simulink model "nms_3Dmodel_inv_wAnkleCPG"  (R2016b)
settings: Solver=ode3  StartTime=0.0  StopTime=tend  FixedStep=ts  RelTol=1e-3  EnableMultiTasking=on
InitFcn:
  | runScripts_inv;
values from neighbouring files (symbols this model uses):
  c = 0.05    [IID_nms_MechInit.m]    (also in nms_MechInit.m)
  c_jointstop = 0.3 / (pi/180)    (= 17.1887338539)    [IID_nms_MechInit.m]    (also in nms_MechInit.m)
  CPG_On = 1    [setCPGPar.m]    (also in setCPGPar_inv.m)
  CtrlPar_FP = [alpha0 alpha_cd alpha_cv]    [setCtrlPar.m]
  CtrlPar_FP_R = [R_hipR0 R_hipR_cd R_hipR_cv]    [setCtrlPar.m]
  CtrlPar_LL = l_clr    [setCtrlPar.m]
  CtrlPar_St = [StPreStim St_M1 St_M2 St_M3 St_M4 St_M5 St_M11]    [setCtrlPar.m]
  CtrlPar_St_R = [R_StPreStim R_St_M1 R_St_M3 R_St_M4]    [setCtrlPar.m]
  CtrlPar_Sw = [SwPreStim SwPhasePari SwPhaseParii SwCtrlPar_H SwCtrlPar_A      SwCtrlPar_Ki SwCtrlPar_Kii SwCtrlPar_Kiii SwCtrlPar_StP]    [setCtrlPar.m]
  CtrlPar_Sw_R = [R_SwPreStim R_Sw_M6]    [setCtrlPar.m]
  CtrlPar_theta0 = parBlCtrl(1)      *1*pi/180    [setCtrlPar.m]
  CtrlPar_Tr = [Tr_St_sup Tr_Sw]    [setCtrlPar.m]
  CtrlPar_Tr_R = [R_Tr_St_sup R_Tr_Sw]    [setCtrlPar.m]
  eref = 0.04    [IID_nms_MechInit.m]    (also in nms_MechInit.m)
  FmaxBFSH = 350    [nms_MechInit.m]
  FmaxGAS = 1500    [IID_nms_MechInit.m]    (also in nms_MechInit.m)
  FmaxGLU = 1500    [IID_nms_MechInit.m]    (also in nms_MechInit.m)
  FmaxHAB = 3000    [nms_MechInit.m]
  FmaxHAD = 4500    [nms_MechInit.m]
  FmaxHAM = 3000    [IID_nms_MechInit.m]    (also in nms_MechInit.m)
  FmaxHFL = 2000    [IID_nms_MechInit.m]    (also in nms_MechInit.m)
  FmaxRF = 1200    [nms_MechInit.m]
  FmaxSOL = 4000    [IID_nms_MechInit.m]    (also in nms_MechInit.m)
  FmaxTA = 800    [IID_nms_MechInit.m]    (also in nms_MechInit.m)
  FmaxVAS = 6000    [IID_nms_MechInit.m]    (also in nms_MechInit.m)
  init_a_tgt = 70*pi/180    (= 1.2217304764)    [setInitPar.m]
  init_a_tgtR = 90*pi/180    (= 1.57079632679)    [setInitPar.m]
  K = 5    [IID_nms_MechInit.m]    (also in nms_MechInit.m)
  leg_l = [D12_T D12_S]    [nms_MechInit.m]
  LongDelay = 0.020    (= 0.02)    [IID_setCtrlPar.m]    (also in nms_MechInit.m = 0.01)
  LongLoopDelay = 0.030    (= 0.03)    [nms_MechInit.m]
  loptBFSH = 0.12    [nms_MechInit.m]
  loptGAS = 0.05    [IID_nms_MechInit.m]    (also in nms_MechInit.m)
  loptGLU = 0.11    [IID_nms_MechInit.m]    (also in nms_MechInit.m)
  loptHAB = 0.09    [nms_MechInit.m]
  loptHAD = 0.10    (= 0.1)    [nms_MechInit.m]
  loptHAM = 0.10    (= 0.1)    [IID_nms_MechInit.m]    (also in nms_MechInit.m)
  loptHFL = 0.11    [IID_nms_MechInit.m]    (also in nms_MechInit.m)
  loptRF = 0.08    [nms_MechInit.m]
  loptSOL = 0.04    [IID_nms_MechInit.m]    (also in nms_MechInit.m)
  loptTA = 0.06    [IID_nms_MechInit.m]    (also in nms_MechInit.m)
  loptVAS = 0.08    [IID_nms_MechInit.m]    (also in nms_MechInit.m)
  lslackBFSH = 0.10    (= 0.1)    [nms_MechInit.m]
  lslackGAS = 0.40    (= 0.4)    [IID_nms_MechInit.m]    (also in nms_MechInit.m)
  lslackGLU = 0.13    [IID_nms_MechInit.m]    (also in nms_MechInit.m)
  lslackHAB = 0.07    [nms_MechInit.m]
  lslackHAD = 0.18    [nms_MechInit.m]
  lslackHAM = 0.31    [IID_nms_MechInit.m]    (also in nms_MechInit.m)
  lslackHFL = 0.10    (= 0.1)    [IID_nms_MechInit.m]    (also in nms_MechInit.m)
  lslackRF = 0.35    [nms_MechInit.m]
  lslackSOL = 0.26    [IID_nms_MechInit.m]    (also in nms_MechInit.m)
  lslackTA = 0.24    [IID_nms_MechInit.m]    (also in nms_MechInit.m)
  lslackVAS = 0.23    [IID_nms_MechInit.m]    (also in nms_MechInit.m)
  massBFSH = 2    [nms_MechInit.m]
  massGAS = 0.45    [IID_nms_MechInit.m]    (also in nms_MechInit.m)
  massGLU = 1.4    [IID_nms_MechInit.m]    (also in nms_MechInit.m)
  massHAB = 1.145    [nms_MechInit.m]
  massHAD = 1.91    [nms_MechInit.m]
  massHAM = 1.82    [IID_nms_MechInit.m]    (also in nms_MechInit.m)
  massHFL = 1.87    [IID_nms_MechInit.m]    (also in nms_MechInit.m)
  massRF = 1    [nms_MechInit.m]
  massSOL = 1.36    [IID_nms_MechInit.m]    (also in nms_MechInit.m)
  massTA = 0.29    [IID_nms_MechInit.m]    (also in nms_MechInit.m)
  massVAS = 2.91    [IID_nms_MechInit.m]    (also in nms_MechInit.m)
  MidDelay = 0.010    (= 0.01)    [IID_setCtrlPar.m]    (also in nms_MechInit.m = 0.005)
  N = 1.5    [IID_nms_MechInit.m]    (also in cmaes_parfor.m = size(x,1); nms_MechInit.m)
  phi12_LowLimit = 70*pi/180    (= 1.2217304764)    [IID_nms_MechInit.m]    (also in nms_MechInit.m)
  phi12_UpLimit = 130*pi/180    (= 2.26892802759)    [IID_nms_MechInit.m]    (also in nms_MechInit.m)
  phi23_UpLimit = 175*pi/180    (= 3.05432619099)    [IID_nms_MechInit.m]    (also in nms_MechInit.m)
  phi34_UpLimit = 230*pi/180    (= 4.01425727959)    [IID_nms_MechInit.m]    (also in nms_MechInit.m)
  phi34R_LowLimit = -15*pi/180    (= -0.261799387799)    [nms_MechInit.m]
  phi34R_UpLimit = 50*pi/180    (= 0.872664625997)    [nms_MechInit.m]
  phimaxGASa = 110*pi/180    (= 1.91986217719)    [IID_nms_MechInit.m]    (also in nms_MechInit.m = 1.74532925199)
  phimaxGASk = 140*pi/180    (= 2.44346095279)    [IID_nms_MechInit.m]    (also in nms_MechInit.m)
  phimaxRFk = 165*pi/180    (= 2.87979326579)    [nms_MechInit.m]
  phimaxSOL = 110*pi/180    (= 1.91986217719)    [IID_nms_MechInit.m]    (also in nms_MechInit.m = 1.74532925199)
  phimaxTA = 80*pi/180    (= 1.3962634016)    [IID_nms_MechInit.m]    (also in nms_MechInit.m)
  phimaxVAS = 165*pi/180    (= 2.87979326579)    [IID_nms_MechInit.m]    (also in nms_MechInit.m)
  phirefBFSH = 160*pi/180    (= 2.79252680319)    [nms_MechInit.m]
  phirefGASa = 80*pi/180    (= 1.3962634016)    [IID_nms_MechInit.m]    (also in nms_MechInit.m)
  phirefGASk = 165*pi/180    (= 2.87979326579)    [IID_nms_MechInit.m]    (also in nms_MechInit.m)
  phirefGLU = 150*pi/180    (= 2.61799387799)    [IID_nms_MechInit.m]    (also in nms_MechInit.m = 2.09439510239)
  phirefHAB = 10*pi/180    (= 0.174532925199)    [nms_MechInit.m]
  phirefHAD = 15*pi/180    (= 0.261799387799)    [nms_MechInit.m]
  phirefHAMh = 155*pi/180    (= 2.70526034059)    [IID_nms_MechInit.m]    (also in nms_MechInit.m = 2.61799387799)
  phirefHAMk = 180*pi/180    (= 3.14159265359)    [IID_nms_MechInit.m]    (also in nms_MechInit.m)
  phirefHFL = 180*pi/180    (= 3.14159265359)    [IID_nms_MechInit.m]    (also in nms_MechInit.m = 2.79252680319)
  phirefRFh = 170*pi/180    (= 2.96705972839)    [nms_MechInit.m]
  phirefRFk = 125*pi/180    (= 2.18166156499)    [nms_MechInit.m]
  phirefSOL = 80*pi/180    (= 1.3962634016)    [IID_nms_MechInit.m]    (also in nms_MechInit.m = 1.57079632679)
  phirefTA = 110*pi/180    (= 1.91986217719)    [IID_nms_MechInit.m]    (also in nms_MechInit.m)
  phirefVAS = 125*pi/180    (= 2.18166156499)    [IID_nms_MechInit.m]    (also in nms_MechInit.m = 2.09439510239)
  phiScaleGASa = acos(rGASamin/rGASamax)/(phiminGASa-phimaxGASa)    [nms_MechInit.m]
  phiScaleGASk = acos(rGASkmin/rGASkmax)/(phiminGASk-phimaxGASk)    [nms_MechInit.m]
  phiScaleRFk = acos(rRFkmin/rRFkmax)/(phiminRFk-phimaxRFk)    [nms_MechInit.m]
  phiScaleSOL = acos(rSOLmin/rSOLmax)/(phiminSOL-phimaxSOL)    [nms_MechInit.m]
  phiScaleTA = acos(rTAmin/rTAmax)/(phiminTA-phimaxTA)    [nms_MechInit.m]
  phiScaleVAS = acos(rVASmin/rVASmax)/(phiminVAS-phimaxVAS)    [nms_MechInit.m]
  rBFSH = 0.04    [nms_MechInit.m]
  rGASamax = 0.06    [nms_MechInit.m]
  rGASkmax = 0.05    [nms_MechInit.m]
  rGLU = 0.10    (= 0.1)    [IID_nms_MechInit.m]    (also in nms_MechInit.m = 0.08)
  rHAB = 0.06    [nms_MechInit.m]
  rHAD = 0.03    [nms_MechInit.m]
  rHAMh = 0.08    [IID_nms_MechInit.m]    (also in nms_MechInit.m)
  rHAMk = 0.05    [IID_nms_MechInit.m]    (also in nms_MechInit.m)
  rHFL = 0.10    (= 0.1)    [IID_nms_MechInit.m]    (also in nms_MechInit.m = 0.08)
  rhoBFSH = 0.7    [nms_MechInit.m]
  rhoGASa = 0.7    [IID_nms_MechInit.m]    (also in nms_MechInit.m)
  rhoGASk = 0.7    [IID_nms_MechInit.m]    (also in nms_MechInit.m)
  rhoGLU = 0.5    [IID_nms_MechInit.m]    (also in nms_MechInit.m)
  rhoHAB = 0.7    [nms_MechInit.m]
  rhoHAD = 1    [nms_MechInit.m]
  rhoHAMh = 0.7    [IID_nms_MechInit.m]    (also in nms_MechInit.m = 0.5)
  rhoHAMk = 0.7    [IID_nms_MechInit.m]    (also in nms_MechInit.m = 0.5)
  rhoHFL = 0.5    [IID_nms_MechInit.m]    (also in nms_MechInit.m)
  rhoRFh = 0.3    [nms_MechInit.m]
  rhoRFk = 0.5    [nms_MechInit.m]
  rhoSOL = 0.5    [IID_nms_MechInit.m]    (also in nms_MechInit.m)
  rhoTA = 0.7    [IID_nms_MechInit.m]    (also in nms_MechInit.m)
  ... (+55 more)
libraries: simulink_extras x30, nmc x30, simulink x22, NMCCPG_Library x13, powerlib_meascontrol x5
(part 2 of 12)

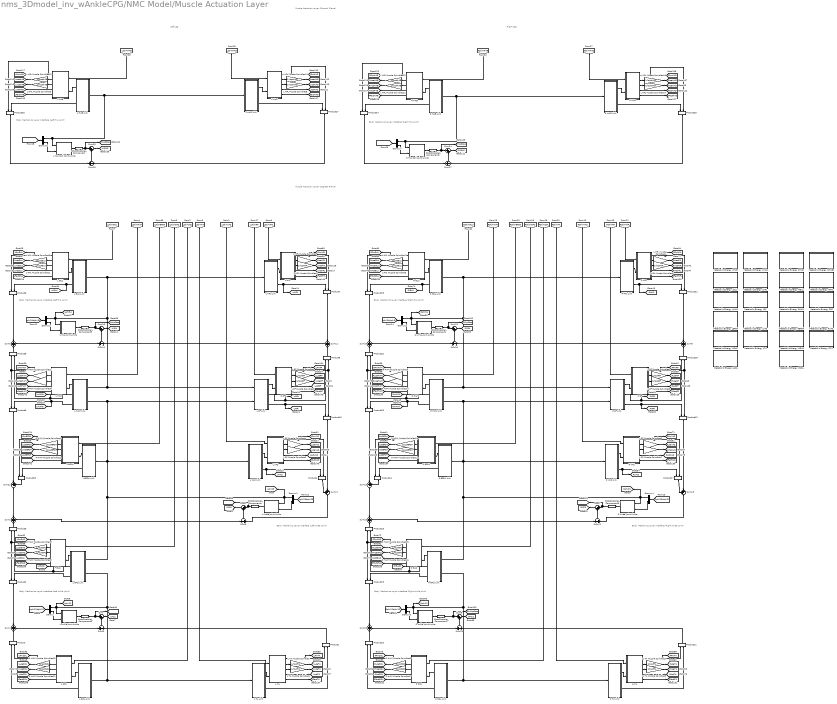
== system nms_3Dmodel_inv_wAnkleCPG/NMC Model/Muscle Actuation Layer ==
  note: Muscle Actuation Layer
      | (Coronal Plane)
  note: Right Leg
  note: Body Mechanics Layer
      | Interface (Right Hip Joint)
  note: Body Mechanics Layer
      | Interface (Left Hip Joint)
  note: Left Leg
  note: Body Mechanics Layer
      | Interface (Right Ankle Joint)
  note: Body Mechanics Layer
      | Interface (Right Knee Joint)
  note: Body Mechanics Layer
      | Interface (Right Hip Joint)
  note: Body Mechanics Layer
      | Interface (Left Ankle Joint)
  note: Body Mechanics Layer
      | Interface (Left Knee Joint)
  note: Body Mechanics Layer
      | Interface (Left Hip Joint)
  note: Muscle Actuation Layer
      | (Sagittal Plane)
  Demux{,1..7} (8 alike) : Demux  Outputs=2
  F GAS : Subsystem
  GotoDisabler_Component{,1..7} (8 alike) : nmc/GotoDisabler_Component  GotoTag=DisableNMC_JointLimits
  L Ankle Joint Limits : Subsystem
  L BFSH : Subsystem
  L BFSH Link : Subsystem
  L GAS Link : Subsystem
  L GLU : Subsystem
  L GLU Link : Subsystem
  L HAB : Subsystem
  L HAB Link : Subsystem
  L HAD : Subsystem
  L HAD Link : Subsystem
  L HAM : Subsystem
  L HAM Link : Subsystem
  L HFL : Subsystem
  L HFL Muscle Spindles{,1,4..5} (4 alike) : Gain  Gain=1/loptHFL
  L HFL Muscle Spindles{9..10,12..13} (4 alike) : Gain  Gain=1/loptHAB
  L HFL Muscle Spindles{8,11,14..15} (4 alike) : Gain  Gain=1/loptHAD
  L HFL Muscle Spindles{2..3,6..7} (4 alike) : Gain  Gain=1/loptGLU
  L HFL Link : Subsystem
  L Hip Joint Limits : Subsystem
  L Hip Roll Joint Limits : Subsystem
  L Knee Joint Limits : Subsystem
  L RF Muscle Spindles{,1..3} (4 alike) : Gain  Gain=1/loptRF
  L RF Muscle Spindles{4..7} (4 alike) : Gain  Gain=1/loptVAS
  L RF Link : Subsystem
  L SOL : Subsystem
  L SOL Link : Subsystem
  L TA : Subsystem
  L TA Muscle Spindles{,1..3} (4 alike) : Gain  Gain=1/loptTA
  L TA Link : Subsystem
  L VAS : Subsystem
  L VAS Link : Subsystem
  Metabolic Energy LBFSH : Subsystem  mask{side='L', muscle='BFSH'}
      mask prompts: side "What Side (R/L)?"; muscle "What Muscle?"
      mask init:
      | blk = gcb;
      | 
      | set_param([gcb '/From1'],'GotoTag',[side,'Act',muscle]);
      | set_param([gcb '/From2'],'GotoTag',[side,'Stim',muscle]);
      | set_param([gcb '/From3'],'GotoTag',[side,'Lce',muscle]);
      | set_param([gcb '/From4'],'GotoTag',[side,'Vce',muscle]);
      | set_param([gcb '/From5'],'GotoTag',[side,'Fm',muscle]);
      | set_param([gcb '/From6'],'GotoTag',[side,'Fact',muscle]);
      | 
      | set_param([gcb '/Goto1'],'GotoTag',[side,'Energy',muscle]);
      | 
      | set_param([gcb '/Constant'],'Value',['lopt',muscle]);
      | set_param([gcb '/Constant1'],'Value',['mass',muscle]);
      | set_param([gcb '/Constant2'],'Value',['t1f',muscle]);
  Metabolic Energy LGAS : Subsystem  mask{side='L', muscle='GAS'}
      mask prompts: side "What Side (R/L)?"; muscle "What Muscle?"
      mask init: same as nms_3Dmodel_inv_wAnkleCPG/NMC Model/Muscle Actuation Layer/Metabolic Energy LBFSH
  Metabolic Energy LGLU : Subsystem  mask{side='L', muscle='GLU'}
      mask prompts: side "What Side (R/L)?"; muscle "What Muscle?"
      mask init: same as nms_3Dmodel_inv_wAnkleCPG/NMC Model/Muscle Actuation Layer/Metabolic Energy LBFSH
  Metabolic Energy LHAB : Subsystem  mask{side='L', muscle='HAB'}
      mask prompts: side "What Side (R/L)?"; muscle "What Muscle?"
      mask init: same as nms_3Dmodel_inv_wAnkleCPG/NMC Model/Muscle Actuation Layer/Metabolic Energy LBFSH
  Metabolic Energy LHAD : Subsystem  mask{side='L', muscle='HAD'}
      mask prompts: side "What Side (R/L)?"; muscle "What Muscle?"
      mask init: same as nms_3Dmodel_inv_wAnkleCPG/NMC Model/Muscle Actuation Layer/Metabolic Energy LBFSH
  Metabolic Energy LHAM : Subsystem  mask{side='L', muscle='HAM'}
      mask prompts: side "What Side (R/L)?"; muscle "What Muscle?"
      mask init: same as nms_3Dmodel_inv_wAnkleCPG/NMC Model/Muscle Actuation Layer/Metabolic Energy LBFSH
  Metabolic Energy LHFL : Subsystem  mask{side='L', muscle='HFL'}
      mask prompts: side "What Side (R/L)?"; muscle "What Muscle?"
      mask init: same as nms_3Dmodel_inv_wAnkleCPG/NMC Model/Muscle Actuation Layer/Metabolic Energy LBFSH
  Metabolic Energy LRF : Subsystem  mask{side='L', muscle='RF'}
      mask prompts: side "What Side (R/L)?"; muscle "What Muscle?"
      mask init: same as nms_3Dmodel_inv_wAnkleCPG/NMC Model/Muscle Actuation Layer/Metabolic Energy LBFSH
  Metabolic Energy LSOL : Subsystem  mask{side='L', muscle='SOL'}
      mask prompts: side "What Side (R/L)?"; muscle "What Muscle?"
      mask init: same as nms_3Dmodel_inv_wAnkleCPG/NMC Model/Muscle Actuation Layer/Metabolic Energy LBFSH
  Metabolic Energy LTA : Subsystem  mask{side='L', muscle='TA'}
      mask prompts: side "What Side (R/L)?"; muscle "What Muscle?"
      mask init: same as nms_3Dmodel_inv_wAnkleCPG/NMC Model/Muscle Actuation Layer/Metabolic Energy LBFSH
  Metabolic Energy LVAS : Subsystem  mask{side='L', muscle='VAS'}
      mask prompts: side "What Side (R/L)?"; muscle "What Muscle?"
      mask init: same as nms_3Dmodel_inv_wAnkleCPG/NMC Model/Muscle Actuation Layer/Metabolic Energy LBFSH
  Metabolic Energy RBFSH : Subsystem  mask{side='R', muscle='BFSH'}
      mask prompts: side "What Side (R/L)?"; muscle "What Muscle?"
      mask init: same as nms_3Dmodel_inv_wAnkleCPG/NMC Model/Muscle Actuation Layer/Metabolic Energy LBFSH
  Metabolic Energy RGAS : Subsystem  mask{side='R', muscle='GAS'}
      mask prompts: side "What Side (R/L)?"; muscle "What Muscle?"
      mask init: same as nms_3Dmodel_inv_wAnkleCPG/NMC Model/Muscle Actuation Layer/Metabolic Energy LBFSH
  Metabolic Energy RGLU : Subsystem  mask{side='R', muscle='GLU'}
      mask prompts: side "What Side (R/L)?"; muscle "What Muscle?"
      mask init: same as nms_3Dmodel_inv_wAnkleCPG/NMC Model/Muscle Actuation Layer/Metabolic Energy LBFSH
  Metabolic Energy RHAB : Subsystem  mask{side='R', muscle='HAB'}
      mask prompts: side "What Side (R/L)?"; muscle "What Muscle?"
      mask init: same as nms_3Dmodel_inv_wAnkleCPG/NMC Model/Muscle Actuation Layer/Metabolic Energy LBFSH
  Metabolic Energy RHAB1 : Subsystem  mask{side='R', muscle='HAD'}
      mask prompts: side "What Side (R/L)?"; muscle "What Muscle?"
      mask init: same as nms_3Dmodel_inv_wAnkleCPG/NMC Model/Muscle Actuation Layer/Metabolic Energy LBFSH
  Metabolic Energy RHAM : Subsystem  mask{side='R', muscle='HAM'}
      mask prompts: side "What Side (R/L)?"; muscle "What Muscle?"
      mask init: same as nms_3Dmodel_inv_wAnkleCPG/NMC Model/Muscle Actuation Layer/Metabolic Energy LBFSH
  Metabolic Energy RHFL : Subsystem  mask{side='R', muscle='HFL'}
      mask prompts: side "What Side (R/L)?"; muscle "What Muscle?"
      mask init: same as nms_3Dmodel_inv_wAnkleCPG/NMC Model/Muscle Actuation Layer/Metabolic Energy LBFSH
  Metabolic Energy RRF : Subsystem  mask{side='R', muscle='RF'}
      mask prompts: side "What Side (R/L)?"; muscle "What Muscle?"
      mask init: same as nms_3Dmodel_inv_wAnkleCPG/NMC Model/Muscle Actuation Layer/Metabolic Energy LBFSH
  Metabolic Energy RSOL : Subsystem  mask{side='R', muscle='SOL'}
      mask prompts: side "What Side (R/L)?"; muscle "What Muscle?"
      mask init: same as nms_3Dmodel_inv_wAnkleCPG/NMC Model/Muscle Actuation Layer/Metabolic Energy LBFSH
  Metabolic Energy RTA : Subsystem  mask{side='R', muscle='TA'}
      mask prompts: side "What Side (R/L)?"; muscle "What Muscle?"
      mask init: same as nms_3Dmodel_inv_wAnkleCPG/NMC Model/Muscle Actuation Layer/Metabolic Energy LBFSH
  Metabolic Energy RVAS : Subsystem  mask{side='R', muscle='VAS'}
      mask prompts: side "What Side (R/L)?"; muscle "What Muscle?"
      mask init: same as nms_3Dmodel_inv_wAnkleCPG/NMC Model/Muscle Actuation Layer/Metabolic Energy LBFSH
  Product{,1..27} (28 alike) : Product  RndMeth=Zero
  R Ankle Joint Limits : Subsystem
  R BFSH : Subsystem
  R BFSH Link : Subsystem
  R GAS : Subsystem
  R GAS Link : Subsystem
  R GLU : Subsystem
  R GLU Link : Subsystem
  R HAB : Subsystem
  R HAB Link : Subsystem
  R HAD : Subsystem
  R HAD Link : Subsystem
  R HAM : Subsystem
  R HAM Muscle Spindles{1,3,6,14} (4 alike) : Gain  Gain=1/loptHAM
  R HAM Muscle Spindles{5,7,10..11} (4 alike) : Gain  Gain=1/loptSOL
  R HAM Muscle Spindles{2,4,12..13} (4 alike) : Gain  Gain=1/loptBFSH
  R HAM Muscle Spindles{8..9,15..16} (4 alike) : Gain  Gain=1/loptGAS
  R HAM Link : Subsystem
  R HFL : Subsystem
  R HFL Link : Subsystem
  R Hip Roll Joint Limits : Subsystem
  R Knee Joint Limits : Subsystem
  R L Hip Joint Limits : Subsystem
  R RF : Subsystem
  R RF Link : Subsystem
  R RF1 : Subsystem
  R SOL : Subsystem
  R SOL Link : Subsystem
  R TA : Subsystem
  R TA Link : Subsystem
  R VAS : Subsystem
  R VAS Link : Subsystem
  Sum{,1,6..7,12,16,18,22,24,26} (10 alike) : Sum  Inputs=|++
  Sum{9..10,14,23,25,27} (6 alike) : Sum  Inputs=+-
  Sum{2..4,8,11,15,19..20} (8 alike) : Sum
  Sum13 : Sum  Inputs=++|
  Sum17 : Sum  Inputs=++|
  Sum21 : Sum  Inputs=-+
  Sum5 : Sum  Inputs=-+
  tag scope: LActBFSH=global, LActGAS=global, LActGLU=global, LActHAB=global, LActHAD=global, LActHAM=global, LActHFL=global, LActRF=global, LActSOL=global, LActTA=global, LActVAS=global, LAnkleStop=global, LFactBFSH=global, LFactGAS=global, LFactGLU=global, LFactHAB=global, LFactHAD=global, LFactHAM=global, LFactHFL=global, LFactRF=global, LFactSOL=global, LFactTA=global, LFactVAS=global, LFmBFSH=global, LFmGAS=global, LFmGLU=global, LFmHAB=global, LFmHAD=global, LFmHAM=global, LFmHFL=global, LFmRF=global, LFmSOL=global, LFmTA=global, LFmVAS=global, LHipRStop=global, LHipStop=global, LKneeStop=global, LLceBFSH=global, LLceGAS=global, LLceGLU=global, LLceHAB=global, LLceHAD=global, LLceHAM=global, LLceHFL=global, LLceRF=global, LLceSOL=global, LLceTA=global, LLceVAS=global, LM12=global, LM23=global, LM34=global, LM34R=global, LVceBFSH=global, LVceGAS=global, LVceGLU=global, LVceHAB=global, LVceHAD=global, LVceHAM=global, LVceHFL=global, LVceRF=global, LVceSOL=global, LVceTA=global, LVceVAS=global, Lphi12=global, Lphi23=global, Lphi34=global, LrGASk=global, LrGLU=global, LrHAMh=global, LrHAMk=global, LrHFL=global, LrRFh=global, LrRFk=global, LrVAS=global, RActBFSH=global, RActGAS=global, RActGLU=global, RActHAB=global, RActHAD=global, RActHAM=global, RActHFL=global, RActRF=global, RActSOL=global, RActTA=global, RActVAS=global, RAnkleStop=global, RFactBFSH=global, RFactGAS=global, RFactGLU=global, RFactHAB=global, RFactHAD=global, RFactHAM=global, RFactHFL=global, RFactRF=global, RFactSOL=global, RFactTA=global, RFactVAS=global, RFmBFSH=global, RFmGAS=global, RFmGLU=global, RFmHAB=global, RFmHAD=global, RFmHAM=global, RFmHFL=global, RFmRF=global, RFmSOL=global, RFmTA=global, RFmVAS=global, RHipStop=global, RHipStopR=global, RKneeStop=global, RLceBFSH=global, RLceGAS=global, RLceGLU=global, RLceHAB=global, RLceHAD=global, RLceHAM=global, RLceHFL=global, RLceRF=global, RLceSOL=global, RLceTA=global, RLceVAS=global, RM12=global, RM23=global, RM34=global, RM34R=global, RVceBFSH=global, RVceGAS=global, RVceGLU=global, RVceHAB=global, RVceHAD=global, RVceHAM=global, RVceHFL=global, RVceRF=global, RVceSOL=global, RVceTA=global, RVceVAS=global, Rphi12=global, Rphi23=global, Rphi34=global, RrGASk=global, RrGLU=global, RrHAMh=global, RrHAMk=global, RrHFL=global, RrRFh=global, RrRFk=global, RrVAS=global
  wires:
  L HAD/5(Fac) -> [LFactHAD]
  L HAB/5(Fac) -> [LFactHAB]
  L GLU/5(Fac) -> [LFactGLU]
  L HFL/5(Fac) -> [LFactHFL]
  R RF1/5(Fac) -> [LFactRF]
  L HAM/5(Fac) -> [LFactHAM]
  L BFSH/5(Fac) -> [LFactBFSH]
  L VAS/5(Fac) -> [LFactVAS]
  F GAS/5(Fac) -> [LFactGAS]
  L SOL/5(Fac) -> [LFactSOL]
  L TA/5(Fac) -> [LFactTA]
  R GLU/5(Fac) -> [RFactGLU]
  R HAM/5(Fac) -> [RFactHAM]
  R BFSH/5(Fac) -> [RFactBFSH]
  R GAS/5(Fac) -> [RFactGAS]
  R SOL/5(Fac) -> [RFactSOL]
  R TA/5(Fac) -> [RFactTA]
  R VAS/5(Fac) -> [RFactVAS]
  R RF/5(Fac) -> [RFactRF]
  R HAB/5(Fac) -> [RFactHAB]
  R HAD/5(Fac) -> [RFactHAD]
  R HFL/5(Fac) -> [RFactHFL]
  R HAD/1(Fmtc) -> Product25/2, [RFmHAD]
  R HAD/4(A) -> [RActHAD]
  R HAD/3(Vce) -> L HFL Muscle Spindles14/1
  R HAD/2(Lce) -> L HFL Muscle Spindles15/1
  L HFL Muscle Spindles15/1 -> [RLceHAD]
  L HFL Muscle Spindles14/1 -> [RVceHAD]
  R HAB/1(Fmtc) -> Product24/1, [RFmHAB]
  L HFL Muscle Spindles13/1 -> [RLceHAB]
  L HFL Muscle Spindles12/1 -> [RVceHAB]
  R HAB/3(Vce) -> L HFL Muscle Spindles12/1
  R HAB/2(Lce) -> L HFL Muscle Spindles13/1
  R HAB/4(A) -> [RActHAB]
  L HAD/1(Fmtc) -> [LFmHAD], Product27/2
  L HAD/4(A) -> [LActHAD]
  L HAD/3(Vce) -> L HFL Muscle Spindles8/1
  L HAD/2(Lce) -> L HFL Muscle Spindles11/1
  L HFL Muscle Spindles11/1 -> [LLceHAD]
  L HFL Muscle Spindles8/1 -> [LVceHAD]
  L HAB/1(Fmtc) -> [LFmHAB], Product26/1
  L HFL Muscle Spindles10/1 -> [LLceHAB]
  L HFL Muscle Spindles9/1 -> [LVceHAB]
  L HAB/3(Vce) -> L HFL Muscle Spindles9/1
  L HAB/2(Lce) -> L HFL Muscle Spindles10/1
  L HAB/4(A) -> [LActHAB]
  [RStimHAB] -> R HAB/1(STIM)
  R HAD Link/2(lever [m]) -> Product25/1
  R HAD Link/1(lmtu [m]) -> R HAD/2(lmtc [m])
  Product25/1 -> Sum27/2
  Sum27/1 -> Sum24/2
  R Hip Roll Joint Limits/1(M_stop [Nm]) -> GotoDisabler_Component2/1
  Demux7/2 -> R Hip Roll Joint Limits/2(dphi [rad/s])
  R HAB Link/2(lever [m]) -> Product24/2
  R HAB Link/1(lmtu [m]) -> R HAB/2(lmtc [m])
  Product24/1 -> Sum27/1
  Demux7/1 -> R Hip Roll Joint Limits/1(phi [rad]), R HAB Link/1(phi34R [rad]), R HAD Link/1(phi34R [rad])
  [Rphi34dphi34R] -> Demux7/1
  Sum24/1 -> [RM34R]
  [RStimHAD] -> R HAD/1(STIM)
  L HAD Link/2(lever [m]) -> Product27/1
  L HAD Link/1(lmtu [m]) -> L HAD/2(lmtc [m])
  Product27/1 -> Sum25/2
  L Hip Roll Joint Limits/1(M_stop [Nm]) -> GotoDisabler_Component/1
  Demux6/2 -> L Hip Roll Joint Limits/2(dphi [rad/s])
  L HAB Link/2(lever [m]) -> Product26/2
  L HAB Link/1(lmtu [m]) -> L HAB/2(lmtc [m])
  Product26/1 -> Sum25/1
  Demux6/1 -> L Hip Roll Joint Limits/1(phi [rad]), L HAD Link/1(phi34R [rad]), L HAB Link/1(phi34R [rad])
  [Lphi34dphi34R] -> Demux6/1
  Sum26/1 -> [LM34R]
  [LStimHAB] -> L HAB/1(STIM)
  [LStimHAD] -> L HAD/1(STIM)
  Sum11/1 -> Sum14/2
  L TA Muscle Spindles2/1 -> [RLceTA]
  L RF Muscle Spindles5/1 -> [RLceVAS]
  R HAM Muscle Spindles12/1 -> [RVceBFSH]
  R HAM Muscle Spindles13/1 -> [RLceBFSH]
  L RF Muscle Spindles3/1 -> [RVceRF]
  L RF Muscle Spindles1/1 -> [RLceRF]
  R HAM Muscle Spindles14/1 -> [RVceHAM]
  R HAM Muscle Spindles3/1 -> [RLceHAM]
  L HFL Muscle Spindles4/1 -> [RLceHFL]
  L TA Muscle Spindles3/1 -> [RVceTA]
  R TA/1(Fmtc) -> [RFmTA], Product11/1
  R HAM Muscle Spindles7/1 -> [RVceSOL]
  R HAM Muscle Spindles5/1 -> [RLceSOL]
  R HAM Muscle Spindles16/1 -> [RVceGAS]
  R HAM Muscle Spindles15/1 -> [RLceGAS]
  R BFSH/1(Fmtc) -> [RFmBFSH], Product14/1
  R RF/1(Fmtc) -> [RFmRF], Product12/2, Product18/2
  L RF Muscle Spindles7/1 -> [RVceVAS]
  L HFL Muscle Spindles7/1 -> [RLceGLU]
  L HFL Muscle Spindles6/1 -> [RVceGLU]
  L HFL Muscle Spindles5/1 -> [RVceHFL]
  Product23/1 -> Sum18/1
  Sum18/1 -> Sum15/1
  Product14/1 -> Sum18/2
  R BFSH/3(Vce) -> R HAM Muscle Spindles12/1
  R BFSH/2(Lce) -> R HAM Muscle Spindles13/1
  R BFSH/4(A) -> [RActBFSH]
  R BFSH Link/2(lever [m]) -> Product14/2
  R BFSH Link/1(lmtu [m]) -> R BFSH/2(lmtc [m])
  [RStimBFSH] -> R BFSH/1(STIM)
  Product17/1 -> Sum13/1
  Sum13/1 -> Sum21/2
  Product12/1 -> Sum13/2
  Product18/1 -> Sum8/2
  Product21/1 -> Sum8/1
  Sum8/1 -> Sum10/2
  [RStimRF] -> R RF/1(STIM)
  R RF Link/3(lever23 [m]) -> [RrRFk], Product12/1
  R RF Link/2(lever34 [m]) -> [RrRFh], Product18/1
  R RF Link/1(lmtu [m]) -> R RF/2(lmtc [m])
  R RF/2(Lce) -> L RF Muscle Spindles1/1
  R RF/3(Vce) -> L RF Muscle Spindles3/1
  R RF/4(A) -> [RActRF]
  R HFL/3(Vce) -> L HFL Muscle Spindles5/1
  R VAS/2(Lce) -> L RF Muscle Spindles5/1
  R VAS/3(Vce) -> L RF Muscle Spindles7/1
  R TA/3(Vce) -> L TA Muscle Spindles3/1
  R SOL/3(Vce) -> R HAM Muscle Spindles7/1
  R SOL/2(Lce) -> R HAM Muscle Spindles5/1
  R GAS/2(Lce) -> R HAM Muscle Spindles15/1
  R GAS/3(Vce) -> R HAM Muscle Spindles16/1
  R HAM/3(Vce) -> R HAM Muscle Spindles14/1
  R GLU/3(Vce) -> L HFL Muscle Spindles6/1
  R GLU/2(Lce) -> L HFL Muscle Spindles7/1
  [RStimVAS] -> R VAS/1(STIM)
  R HFL Link/2(lever [m]) -> [RrHFL], Product21/1
  R HFL/4(A) -> [RActHFL]
  R HFL Link/1(lmtu [m]) -> R HFL/2(lmtc [m])
  Sum10/1 -> Sum12/2
  R L Hip Joint Limits/1(M_stop [Nm]) -> GotoDisabler_Component1/1
  Demux5/2 -> R L Hip Joint Limits/2(dphi [rad/s])
  R GLU/4(A) -> [RActGLU]
  R GLU Link/2(lever [m]) -> [RrGLU], Product19/2
  R GLU Link/1(lmtu [m]) -> R GLU/2(lmtc [m])
  Product19/1 -> Sum19/1
  Product22/1 -> Sum19/2
  R HAM/4(A) -> [RActHAM]
  Sum15/1 -> Sum21/1
  R VAS Link/2(lever [m]) -> Product17/1, [RrVAS]
  Sum21/1 -> Sum7/2
  R Knee Joint Limits/1(M_stop [Nm]) -> GotoDisabler_Component5/1
  Sum7/1 -> [RM23]
  R VAS/1(Fmtc) -> [RFmVAS], Product17/2
  R VAS/4(A) -> [RActVAS]
  R GAS/4(A) -> [RActGAS]
  R SOL/4(A) -> [RActSOL]
  Sum6/1 -> [RM12]
  R Ankle Joint Limits/1(M_stop [Nm]) -> GotoDisabler_Component7/1
  Product11/1 -> Sum23/2
  R TA Link/2(lever [m]) -> Product11/2
  Product13/1 -> Sum20/1
  Product10/1 -> Sum20/2
  R SOL Link/2(lever [m]) -> Product10/1
  Demux5/1 -> [Rphi34], R HAM Link/1(phi34 [rad]), R RF Link/1(phi34 [rad]), R GLU Link/1(phi34 [rad]), R HFL Link/1(phi34 [rad]), R L Hip Joint Limits/1(phi [rad])
  [Rphi34dphi34] -> Demux5/1
  [Rphi23dphi23] -> Demux4/1
  [Rphi12dphi12] -> Demux3/1
  Sum20/1 -> Sum23/1
  Sum19/1 -> Sum10/1
  Product16/1 -> Sum15/2
  R HAM Link/3(lever23 [m]) -> [RrHAMk], Product23/2
  R HAM Link/2(lever34 [m]) -> [RrHAMh], Product22/2
  R HAM Link/1(lmtu [m]) -> R HAM/2(lmtc [m])
  R VAS Link/1(lmtu [m]) -> R VAS/2(lmtc [m])
  R GAS Link/1(lmtu [m]) -> R GAS/2(lmtc [m])
  [RStimGAS] -> R GAS/1(STIM)
  R GAS Link/2(lever23 [m]) -> [RrGASk], Product16/2
  R GAS Link/3(lever12 [m]) -> Product13/2
  R TA Link/1(lmtc [m]) -> R TA/2(lmtc [m])
  R SOL Link/1(lmtc [m]) -> R SOL/2(lmtc [m])
  Demux4/2 -> R Knee Joint Limits/2(dphi [rad/s])
  Sum23/1 -> Sum6/2
  Demux3/2 -> R Ankle Joint Limits/2(dphi [rad/s])
  Sum12/1 -> [RM34]
  [RStimGLU] -> R GLU/1(STIM)
  R GLU/1(Fmtc) -> [RFmGLU], Product19/1
  [RStimHFL] -> R HFL/1(STIM)
  R HFL/2(Lce) -> L HFL Muscle Spindles4/1
  R HFL/1(Fmtc) -> [RFmHFL], Product21/2
  R HAM/2(Lce) -> R HAM Muscle Spindles3/1
  R HAM/1(Fmtc) -> [RFmHAM], Product22/1, Product23/1
  [RStimHAM] -> R HAM/1(STIM)
  [RStimSOL] -> R SOL/1(STIM)
  [RStimTA] -> R TA/1(STIM)
  Demux3/1 -> [Rphi12], R Ankle Joint Limits/1(phi [rad]), R GAS Link/2(phi12 [rad]), R TA Link/1(phi12 [rad]), R SOL Link/1(phi12 [rad])
  R GAS/1(Fmtc) -> [RFmGAS], Product16/1, Product13/1
  R TA/4(A) -> [RActTA]
  R TA/2(Lce) -> L TA Muscle Spindles2/1
  R SOL/1(Fmtc) -> [RFmSOL], Product10/2
  Demux4/1 -> [Rphi23], R GAS Link/1(phi23 [rad]), R BFSH Link/1(phi23 [rad]), R HAM Link/2(phi23 [rad]), R RF Link/2(phi23 [rad]), R VAS Link/1(phi23 [rad]), R Knee Joint Limits/1(phi [rad])
  L TA Muscle Spindles/1 -> [LLceTA]
  L RF Muscle Spindles4/1 -> [LLceVAS]
  R HAM Muscle Spindles2/1 -> [LVceBFSH]
  R HAM Muscle Spindles4/1 -> [LLceBFSH]
  L RF Muscle Spindles2/1 -> [LVceRF]
  L RF Muscle Spindles/1 -> [LLceRF]
  R HAM Muscle Spindles6/1 -> [LVceHAM]
  R HAM Muscle Spindles1/1 -> [LLceHAM]
  L HFL Muscle Spindles/1 -> [LLceHFL]
  L TA Muscle Spindles1/1 -> [LVceTA]
  L TA/1(Fmtc) -> Product1/1, [LFmTA]
  R HAM Muscle Spindles11/1 -> [LVceSOL]
  R HAM Muscle Spindles10/1 -> [LLceSOL]
  R HAM Muscle Spindles9/1 -> [LVceGAS]
  R HAM Muscle Spindles8/1 -> [LLceGAS]
  L BFSH/1(Fmtc) -> [LFmBFSH], Product20/1
  R RF1/1(Fmtc) -> Product15/2, Product5/2, [LFmRF]
  L RF Muscle Spindles6/1 -> [LVceVAS]
  L HFL Muscle Spindles3/1 -> [LLceGLU]
  L HFL Muscle Spindles2/1 -> [LVceGLU]
  L HFL Muscle Spindles1/1 -> [LVceHFL]
  Product9/1 -> Sum22/1
  Sum22/1 -> Sum2/1
  Product20/1 -> Sum22/2
  L BFSH/3(Vce) -> R HAM Muscle Spindles2/1
  L BFSH/2(Lce) -> R HAM Muscle Spindles4/1
  L BFSH/4(A) -> [LActBFSH]
  L BFSH Link/2(lever [m]) -> Product20/2
  L BFSH Link/1(lmtu [m]) -> L BFSH/2(lmtc [m])
  [LStimBFSH] -> L BFSH/1(STIM)
  Product4/1 -> Sum17/1
  Sum17/1 -> Sum5/2
  Product15/1 -> Sum17/2
  Product5/1 -> Sum11/2
  Product7/1 -> Sum11/1
  [LStimRF] -> R RF1/1(STIM)
  L RF Link/3(lever23 [m]) -> [LrRFk], Product15/1
  L RF Link/2(lever34 [m]) -> [LrRFh], Product5/1
  L RF Link/1(lmtu [m]) -> R RF1/2(lmtc [m])
  R RF1/2(Lce) -> L RF Muscle Spindles/1
  R RF1/3(Vce) -> L RF Muscle Spindles2/1
  R RF1/4(A) -> [LActRF]
  L HFL/3(Vce) -> L HFL Muscle Spindles1/1
  L VAS/2(Lce) -> L RF Muscle Spindles4/1
  L VAS/3(Vce) -> L RF Muscle Spindles6/1
  L TA/3(Vce) -> L TA Muscle Spindles1/1
  L SOL/3(Vce) -> R HAM Muscle Spindles11/1
  L SOL/2(Lce) -> R HAM Muscle Spindles10/1
  F GAS/2(Lce) -> R HAM Muscle Spindles8/1
  F GAS/3(Vce) -> R HAM Muscle Spindles9/1
  L HAM/3(Vce) -> R HAM Muscle Spindles6/1
  L GLU/3(Vce) -> L HFL Muscle Spindles2/1
  L GLU/2(Lce) -> L HFL Muscle Spindles3/1
  [LStimVAS] -> L VAS/1(STIM)
  L HFL Link/2(lever [m]) -> [LrHFL], Product7/1
  L HFL/4(A) -> [LActHFL]
  L HFL Link/1(lmtu [m]) -> L HFL/2(lmtc [m])
  Sum14/1 -> Sum16/2
  L Hip Joint Limits/1(M_stop [Nm]) -> GotoDisabler_Component3/1
  Demux2/2 -> L Hip Joint Limits/2(dphi [rad/s])
  L GLU/4(A) -> [LActGLU]
  L GLU Link/2(lever [m]) -> [LrGLU], Product6/2
  L GLU Link/1(lmtu [m]) -> L GLU/2(lmtc [m])
  Product6/1 -> Sum3/1
  Product8/1 -> Sum3/2
  L HAM/4(A) -> [LActHAM]
  Sum2/1 -> Sum5/1
  L VAS Link/2(lever [m]) -> Product4/1, [LrVAS]
  Sum5/1 -> Sum1/2
  L Knee Joint Limits/1(M_stop [Nm]) -> GotoDisabler_Component4/1
  Sum1/1 -> [LM23]
  L VAS/1(Fmtc) -> Product4/2, [LFmVAS]
  L VAS/4(A) -> [LActVAS]
  F GAS/4(A) -> [LActGAS]
  L SOL/4(A) -> [LActSOL]
  Sum/1 -> [LM12]
  L Ankle Joint Limits/1(M_stop [Nm]) -> GotoDisabler_Component6/1
  Product1/1 -> Sum9/2
  L TA Link/2(lever [m]) -> Product1/2
  Product2/1 -> Sum4/1
  Product/1 -> Sum4/2
  L SOL Link/2(lever [m]) -> Product/1
  Demux2/1 -> [Lphi34], L HAM Link/1(phi34 [rad]), L RF Link/1(phi34 [rad]), L GLU Link/1(phi34 [rad]), L HFL Link/1(phi34 [rad]), L Hip Joint Limits/1(phi [rad])
  [Lphi34dphi34] -> Demux2/1
  [Lphi23dphi23] -> Demux1/1
  [Lphi12dphi12] -> Demux/1
  Sum4/1 -> Sum9/1
  Sum3/1 -> Sum14/1
  Product3/1 -> Sum2/2
  L HAM Link/3(lever23 [m]) -> [LrHAMk], Product9/2
  L HAM Link/2(lever34 [m]) -> [LrHAMh], Product8/2
  L HAM Link/1(lmtu [m]) -> L HAM/2(lmtc [m])
  L VAS Link/1(lmtu [m]) -> L VAS/2(lmtc [m])
  L GAS Link/1(lmtu [m]) -> F GAS/2(lmtc [m])
  [LStimGAS] -> F GAS/1(STIM)
  L GAS Link/2(lever23 [m]) -> [LrGASk], Product3/2
  L GAS Link/3(lever12 [m]) -> Product2/2
  L TA Link/1(lmtc [m]) -> L TA/2(lmtc [m])
  L SOL Link/1(lmtc [m]) -> L SOL/2(lmtc [m])
  Demux1/2 -> L Knee Joint Limits/2(dphi [rad/s])
  Sum9/1 -> Sum/2
  Demux/2 -> L Ankle Joint Limits/2(dphi [rad/s])
  Sum16/1 -> [LM34]
  [LStimGLU] -> L GLU/1(STIM)
  L GLU/1(Fmtc) -> Product6/1, [LFmGLU]
  [LStimHFL] -> L HFL/1(STIM)
  L HFL/2(Lce) -> L HFL Muscle Spindles/1
  L HFL/1(Fmtc) -> Product7/2, [LFmHFL]
  L HAM/2(Lce) -> R HAM Muscle Spindles1/1
  L HAM/1(Fmtc) -> Product8/1, Product9/1, [LFmHAM]
  [LStimHAM] -> L HAM/1(STIM)
  [LStimSOL] -> L SOL/1(STIM)
  [LStimTA] -> L TA/1(STIM)
  Demux/1 -> [Lphi12], L Ankle Joint Limits/1(phi [rad]), L GAS Link/2(phi12 [rad]), L TA Link/1(phi12 [rad]), L SOL Link/1(phi12 [rad])
  F GAS/1(Fmtc) -> Product3/1, Product2/1, [LFmGAS]
  L TA/4(A) -> [LActTA]
  L TA/2(Lce) -> L TA Muscle Spindles/1
  L SOL/1(Fmtc) -> Product/2, [LFmSOL]
  Demux1/1 -> [Lphi23], L GAS Link/1(phi23 [rad]), L BFSH Link/1(phi23 [rad]), L HAM Link/2(phi23 [rad]), L RF Link/2(phi23 [rad]), L VAS Link/1(phi23 [rad]), L Knee Joint Limits/1(phi [rad])
  GotoDisabler_Component/1 -> [LHipRStop], Sum26/1
  Sum25/1 -> Sum26/2
  GotoDisabler_Component2/1 -> [RHipStopR], Sum24/1
  GotoDisabler_Component1/1 -> [RHipStop], Sum12/1
  GotoDisabler_Component3/1 -> [LHipStop], Sum16/1
  GotoDisabler_Component4/1 -> Sum1/1, [LKneeStop]
  GotoDisabler_Component5/1 -> Sum7/1, [RKneeStop]
  GotoDisabler_Component6/1 -> [LAnkleStop], Sum/1
  GotoDisabler_Component7/1 -> [RAnkleStop], Sum6/1
